simulink model "Q4"  (R2018a)
settings: Solver=VariableStepAuto  StartTime=0.0  StopTime=0.2  MaxStep=1e-2  RelTol=1e-3  AbsTol=1e-3
settings Model: Creator=Kasra  LastModifiedBy=Kasra

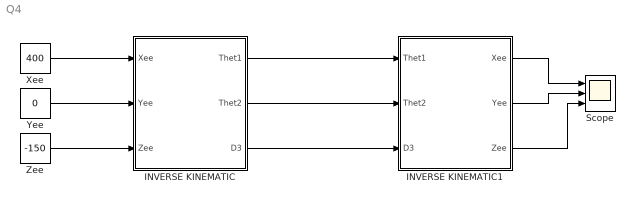
== system Q4 ==
  INVERSE KINEMATIC : MATLAB Function  TreatAsAtomicUnit=on
  INVERSE KINEMATIC1 : MATLAB Function  TreatAsAtomicUnit=on
  Scope : Scope  NumInputPorts=3
  Xee : Constant  Value=400
  Yee : Constant  Value=0
  Zee : Constant  Value=-150
  wires:
  Zee/1 -> INVERSE KINEMATIC/3(Zee)
  Yee/1 -> INVERSE KINEMATIC/2(Yee)
  Xee/1 -> INVERSE KINEMATIC/1(Xee)
  INVERSE KINEMATIC/1(Thet1) -> INVERSE KINEMATIC1/1(Thet1)
  INVERSE KINEMATIC/2(Thet2) -> INVERSE KINEMATIC1/2(Thet2)
  INVERSE KINEMATIC/3(D3) -> INVERSE KINEMATIC1/3(D3)
  INVERSE KINEMATIC1/1(Xee) -> Scope/1
  INVERSE KINEMATIC1/2(Yee) -> Scope/2
  INVERSE KINEMATIC1/3(Zee) -> Scope/3

== matlab function Q4/INVERSE KINEMATIC1 ==
  data: Thet1 input; Xee output; Thet2 input; D3 input; Yee output; Zee output
function [Xee, Yee, Zee] = fcn(Thet1, Thet2, D3)

a1 = 250;
a2 = 150;
d4 = 50;

Xee = a1 * cos(Thet1) + a2 * cos(Thet1 + Thet2);
Yee = a1 * sin(Thet1) + a2 * sin(Thet1 + Thet2);
Zee = -D3 - d4;

end

== matlab function Q4/INVERSE KINEMATIC ==
  data: Xee input; Thet1 output; Yee input; Zee input; Thet2 output; D3 output
function [Thet1, Thet2, D3] = fcn(Xee, Yee, Zee)

coder.extrinsic('solverInverse');
[t1, t2, di3] = solverInverse(Xee, Yee, Zee);
Thet1 = 0;
Thet2 = 0; 
D3 = 0;
Theta1 = min(t1);
Theta2 = min(t2);
D3 = min(di3);
end
